simulink model "Citation_FlightGear_v2"  (R2026a)
settings: Solver=ode5  StopTime=40  FixedStep=0.01  EnableMultiTasking=on
InitFcn:
  | run('initcit.m')
  | run('id_init.m')
values from neighbouring files (symbols this model uses):
  cv1 = 20000    [gear_params.m]
  cv2 = cv1    (= 20000)    [gear_params.m]
  cv3 = 4000    [gear_params.m]
  cv4 = 20000    [gear_params.m]
  deltagmax1 = 0.25    [gear_params.m]
  deltagmax2 = deltagmax1    (= 0.25)    [gear_params.m]
  deltagmax3 = 0.24    [gear_params.m]
  deltagmax4 = 0.02    [gear_params.m]
  kt1 = 525020    [gear_params.m]
  kt2 = kt1    (= 525020)    [gear_params.m]
  kt3 = 457050    [gear_params.m]
  murol = 0.03*10    (= 0.3)    [gear_params.m]
  P1 = 2000    [gear_params.m]
  P2 = P1    (= 2000)    [gear_params.m]
  P3 = 2550    [gear_params.m]
  P4 = 40000    [gear_params.m]
  PL0 = 10000*eye(6)    [id_init.m]
  PM0 = 10000*eye(4)    [id_init.m]
  PN0 = 10000*eye(6)    [id_init.m]
  PX0 = 10000*eye(5)    [id_init.m]
  PY0 = 10000*eye(6)    [id_init.m]
  PZ0 = 10000*eye(4)    [id_init.m]
  thetaL0 = zeros(6,1)    [id_init.m]
  thetaM0 = zeros(4,1)    [id_init.m]
  thetaN0 = zeros(6,1)    [id_init.m]
  thetaX0 = zeros(5,1)    [id_init.m]
  thetaY0 = zeros(6,1)    [id_init.m]
  thetaZ0 = zeros(4,1)    [id_init.m]
  TL = 7.0875e-06    [id_init.m]    (also in plot_comparison_step_4.m = T_var(4))
  TM = 3.2564e-06    [id_init.m]    (also in plot_comparison_step_4.m = T_var(5))
  TN = 5.4692e-07    [id_init.m]    (also in plot_comparison_step_4.m = T_var(6))
  TX = 2.2784e-06    [id_init.m]    (also in plot_comparison_step_4.m = T_var(1))
  TY = 8.0633e-07    [id_init.m]    (also in plot_comparison_step_4.m = T_var(2))
  TZ = 2.8004e-05    [id_init.m]    (also in plot_comparison_step_4.m = T_var(3))
  xl1 = xcg-6.858    [gear_params.m]
  xl2 = xcg-6.858    [gear_params.m]
  xl3 = xcg-2.0752    [gear_params.m]
  xl4 = xcg-12.742    [gear_params.m]
  yl1 = 1.918    [gear_params.m]
  yl2 = -1.918    [gear_params.m]
  yl3 = 0    [gear_params.m]
  yl4 = 0    [gear_params.m]
  zl1 = zcg-1.701    [gear_params.m]
  zl2 = zcg-1.701    [gear_params.m]
  zl3 = zcg-1.7488    [gear_params.m]
  zl4 = zcg-2.78    [gear_params.m]
undefined symbols (not defined in the file or in its folder): chord, Deng, ealphag, ealphas, g0, hDME, hGS, lh, massinit, matbuaf, matdaf, matdam, matdbbf, matdeaf, matdgaf, matdqaf, matduaf, matdwaw, matedhr, mateif, matelhr, matemhr, matemv1, matemv2, matemve, matetam, mateuaf, matfaaf, matfaxl, matff, matibaf, matibb, matibmh, matipaf, matipmh, matiraf, matiuaf, matiwaf, matlaf, matlam, matleaf, matleam, matlgaf, matlqaf, matluaf, matmaaf, matmaam, matmaf, matmam, matmbbf, matmeaf, matmeam, matmgaf, matmqaf, matmrbr, matn1d, matn2d, matnbab, matnbaf, matnbmh ... (+53)
libraries: simulink x12, aerolibfltsims x3, aerolibconvert2 x2, aerolibobsolete x1, aerolibanimutils x1
(part 5 of 5)

== system Citation_FlightGear_v2/Cessna Citation 500/Citation model DASMAT/AIRCRAFT MODEL/EFM/Engmod/Citation eng_mod/Subsystem1/JT15 Dynamic1/Subsystem/engine/Gasgenerator ==
  note: N2 feedback
  note: N2dot
  PBCP : Inport
  he : Inport  Port=2
  sqrt(theta2) : Inport  Port=3
  Droop : Lookup  InputValues=[0 100]  Table="[0.1  2]"
  Fcn : Fcn  Expr=u[1]/u[2]
  Fcn1 : Fcn  Expr=u[1]/u[2]
  Governor : Product  InputSameDT=on  SaturateOnIntegerOverflow=on  OutDataTypeStr=Inherit: Same as first input
  Max accel : Subsystem  mask(Max Value){}
      mask help:
      | Output is maximum value of inputs.
      | y=max(u1,u2)
      mask Help: The Max block produces as output the maximum value of two scalars or vectors. If the inputs are vectors, the output will be a vector containing the maximum elements of the vectors.
      mask Display: disp('Max')
  Min accel : Subsystem  mask(Min Value){}
      mask help:
      | Output is minimum value of inputs.
      | y=min(u1,u2)
      mask Help: The Min block produces as output the minimum value of two scalars or vectors. If the inputs are vectors, the output will be a vector containing the minimum elements of the vectors.
      mask Display: disp('Min')
  Mux : Mux  Inputs=2
  Mux1 : Mux  Inputs=2
  N2 state : Integrator  InitialCondition=xt0(1)
  N2D : Lookup2D  RowIndex=matn2d(2:10,1)  ColumnIndex=matn2d(1,2:10)  Table=matn2d(2:10,2:10)
  Sum : Sum  Inputs=+-  InputSameDT=on  SaturateOnIntegerOverflow=on  OutDataTypeStr=Inherit: Same as first input
  fN2max : Lookup  InputValues=[25 40 70 94]  Table=[0 3 8 10]
  fN2min : Lookup  InputValues="[25     50   60   94 100]"  Table="[-0.05  -0.05    -2    -20 -28]"
  ft2FL : Gain  Gain=.01  SaturateOnIntegerOverflow=on  OutDataTypeStr=Inherit: Same as input  ParamDataTypeStr=Inherit: Same as input
  m2ft : Gain  Gain=(1/0.3048)  SaturateOnIntegerOverflow=on  OutDataTypeStr=Inherit: Same as input  ParamDataTypeStr=Inherit: Same as input
  N2 : Outport
  N2c : Outport  Port=2
  N2cdem : Outport  Port=3
  wires:
  sqrt(theta2)/1 -> Mux1/2, Mux/2
  N2D/1 -> Mux/1, Droop/1, Sum/1
  Fcn1/1 -> N2c/1
  Fcn/1 -> N2cdem/1
  Mux1/1 -> Fcn1/1
  Mux/1 -> Fcn/1
  Min accel/1(out_1) -> Max accel/1(in_1)
  ft2FL/1 -> N2D/2
  m2ft/1 -> ft2FL/1
  he/1 -> m2ft/1
  N2 state/1 -> Mux1/1, fN2min/1, fN2max/1, Sum/2, N2/1
  fN2max/1 -> Min accel/2(in_2)
  fN2min/1 -> Max accel/2(in_2)
  PBCP/1 -> N2D/1
  Droop/1 -> Governor/1
  Sum/1 -> Governor/2
  Governor/1 -> Min accel/1(in_1)
  Max accel/1(out_1) -> N2 state/1

== system Citation_FlightGear_v2/Cessna Citation 500/Citation model DASMAT/AIRCRAFT MODEL/EFM/Engmod/Citation eng_mod/Subsystem1/JT15 Dynamic/Subsystem/engine/Fan/Max accel ==
  in_1 : Inport
  in_2 : Inport  Port=2
  Sum : Sum  Inputs=-+  InputSameDT=on  SaturateOnIntegerOverflow=on  OutDataTypeStr=Inherit: Same as first input
  Switch : Switch
  out_1 : Outport
  wires:
  in_1/1 -> Sum/1, Switch/1
  in_2/1 -> Sum/2, Switch/3
  Sum/1 -> Switch/2
  Switch/1 -> out_1/1

== system Citation_FlightGear_v2/Cessna Citation 500/Citation model DASMAT/AIRCRAFT MODEL/EFM/Engmod/Citation eng_mod/Subsystem1/JT15 Dynamic/Subsystem/engine/Fan/Max decel ==
  in_1 : Inport
  in_2 : Inport  Port=2
  Sum : Sum  Inputs=+-  InputSameDT=on  SaturateOnIntegerOverflow=on  OutDataTypeStr=Inherit: Same as first input
  Switch : Switch
  out_1 : Outport
  wires:
  Switch/1 -> out_1/1
  Sum/1 -> Switch/2
  in_2/1 -> Sum/2, Switch/3
  in_1/1 -> Sum/1, Switch/1

== system Citation_FlightGear_v2/Cessna Citation 500/Citation model DASMAT/AIRCRAFT MODEL/EFM/Engmod/Citation eng_mod/Subsystem1/JT15 Dynamic/Subsystem/engine/Gasgenerator/Max accel ==
  in_1 : Inport
  in_2 : Inport  Port=2
  Sum : Sum  Inputs=+-  InputSameDT=on  SaturateOnIntegerOverflow=on  OutDataTypeStr=Inherit: Same as first input
  Switch : Switch
  out_1 : Outport
  wires:
  Switch/1 -> out_1/1
  Sum/1 -> Switch/2
  in_2/1 -> Sum/2, Switch/3
  in_1/1 -> Sum/1, Switch/1

== system Citation_FlightGear_v2/Cessna Citation 500/Citation model DASMAT/AIRCRAFT MODEL/EFM/Engmod/Citation eng_mod/Subsystem1/JT15 Dynamic/Subsystem/engine/Gasgenerator/Min accel ==
  in_1 : Inport
  in_2 : Inport  Port=2
  Sum : Sum  Inputs=-+  InputSameDT=on  SaturateOnIntegerOverflow=on  OutDataTypeStr=Inherit: Same as first input
  Switch : Switch
  out_1 : Outport
  wires:
  in_1/1 -> Sum/1, Switch/1
  in_2/1 -> Sum/2, Switch/3
  Sum/1 -> Switch/2
  Switch/1 -> out_1/1

== system Citation_FlightGear_v2/Cessna Citation 500/Citation model DASMAT/AIRCRAFT MODEL/EFM/Engmod/Citation eng_mod/Subsystem1/JT15 Dynamic1/Subsystem/engine/Fan/Max accel ==
  in_1 : Inport
  in_2 : Inport  Port=2
  Sum : Sum  Inputs=-+  InputSameDT=on  SaturateOnIntegerOverflow=on  OutDataTypeStr=Inherit: Same as first input
  Switch : Switch
  out_1 : Outport
  wires:
  in_1/1 -> Sum/1, Switch/1
  in_2/1 -> Sum/2, Switch/3
  Sum/1 -> Switch/2
  Switch/1 -> out_1/1

== system Citation_FlightGear_v2/Cessna Citation 500/Citation model DASMAT/AIRCRAFT MODEL/EFM/Engmod/Citation eng_mod/Subsystem1/JT15 Dynamic1/Subsystem/engine/Fan/Max decel ==
  in_1 : Inport
  in_2 : Inport  Port=2
  Sum : Sum  Inputs=+-  InputSameDT=on  SaturateOnIntegerOverflow=on  OutDataTypeStr=Inherit: Same as first input
  Switch : Switch
  out_1 : Outport
  wires:
  Switch/1 -> out_1/1
  Sum/1 -> Switch/2
  in_2/1 -> Sum/2, Switch/3
  in_1/1 -> Sum/1, Switch/1

== system Citation_FlightGear_v2/Cessna Citation 500/Citation model DASMAT/AIRCRAFT MODEL/EFM/Engmod/Citation eng_mod/Subsystem1/JT15 Dynamic1/Subsystem/engine/Gasgenerator/Max accel ==
  in_1 : Inport
  in_2 : Inport  Port=2
  Sum : Sum  Inputs=+-  InputSameDT=on  SaturateOnIntegerOverflow=on  OutDataTypeStr=Inherit: Same as first input
  Switch : Switch
  out_1 : Outport
  wires:
  Switch/1 -> out_1/1
  Sum/1 -> Switch/2
  in_2/1 -> Sum/2, Switch/3
  in_1/1 -> Sum/1, Switch/1

== system Citation_FlightGear_v2/Cessna Citation 500/Citation model DASMAT/AIRCRAFT MODEL/EFM/Engmod/Citation eng_mod/Subsystem1/JT15 Dynamic1/Subsystem/engine/Gasgenerator/Min accel ==
  in_1 : Inport
  in_2 : Inport  Port=2
  Sum : Sum  Inputs=-+  InputSameDT=on  SaturateOnIntegerOverflow=on  OutDataTypeStr=Inherit: Same as first input
  Switch : Switch
  out_1 : Outport
  wires:
  in_1/1 -> Sum/1, Switch/1
  in_2/1 -> Sum/2, Switch/3
  Sum/1 -> Switch/2
  Switch/1 -> out_1/1

== matlab function Citation_FlightGear_v2/RLS for CZ ==
  data: z input; theta_new output; phi input; theta_old input; P_old input; lambda input; reset input; P_new output; yhat output; innovation output
function [theta_new,P_new,yhat,innovation] = ...
    RLS_CZ(z,phi,theta_old,P_old,lambda,reset)

phi = phi(:);

% Previous covariance
Puse = P_old;

% Later used by Step 4
% Reset covariance, not parameter estimate
if reset > 0.5
    n = size(P_old,1);
    Puse = 10000*eye(n);
end

% Prediction using previous parameter estimate
yhat = phi.'*theta_old;

% Innovation
innovation = z - yhat;

% RLS gain
den = lambda + phi.'*Puse*phi;
K = (Puse*phi)/den;

% Parameter update
theta_new = theta_old + K*innovation;

% Covariance update
P_new = (Puse - K*(phi.'*Puse))/lambda;

% Remove numerical asymmetry
P_new = 0.5*(P_new + P_new.');

end

== matlab function Citation_FlightGear_v2/RLS for CL ==
  data: z input; theta_new output; phi input; theta_old input; P_old input; lambda input; reset input; P_new output; yhat output; innovation output
function [theta_new,P_new,yhat,innovation] = ...
    RLS_CL(z,phi,theta_old,P_old,lambda,reset)

phi = phi(:);

% Previous covariance
Puse = P_old;

% Later used by Step 4
% Reset covariance, not parameter estimate
if reset > 0.5
    n = size(P_old,1);
    Puse = 10000*eye(n);
end

% Prediction using previous parameter estimate
yhat = phi.'*theta_old;

% Innovation
innovation = z - yhat;

% RLS gain
den = lambda + phi.'*Puse*phi;
K = (Puse*phi)/den;

% Parameter update
theta_new = theta_old + K*innovation;

% Covariance update
P_new = (Puse - K*(phi.'*Puse))/lambda;

% Remove numerical asymmetry
P_new = 0.5*(P_new + P_new.');

end

== matlab function Citation_FlightGear_v2/RLS for Cm ==
  data: z input; theta_new output; phi input; theta_old input; P_old input; lambda input; reset input; P_new output; yhat output; innovation output
function [theta_new,P_new,yhat,innovation] = ...
    RLS_Cm(z,phi,theta_old,P_old,lambda,reset)

phi = phi(:);

% Previous covariance
Puse = P_old;

% Later used by Step 4
% Reset covariance, not parameter estimate
if reset > 0.5
    n = size(P_old,1);
    Puse = 10000*eye(n);
end

% Prediction using previous parameter estimate
yhat = phi.'*theta_old;

% Innovation
innovation = z - yhat;

% RLS gain
den = lambda + phi.'*Puse*phi;
K = (Puse*phi)/den;

% Parameter update
theta_new = theta_old + K*innovation;

% Covariance update
P_new = (Puse - K*(phi.'*Puse))/lambda;

% Remove numerical asymmetry
P_new = 0.5*(P_new + P_new.');

end

== matlab function Citation_FlightGear_v2/Monitoring/Monitoring Metrics ==
  data: innovations input; MA2 output; AUTOCORR output; VARIANCE output
function [MA2, AUTOCORR, VARIANCE] = monitor_metrics(innovations)
%#codegen

% Number of samples in monitoring window
N = 50;

% Lag used for autocorrelation
kgap = 5;

% Store previous innovation samples
persistent buffer count

if isempty(buffer)
    buffer = zeros(N,6);
    count = 0;
end

% Make sure innovations is a column vector
innovations = innovations(:);

% ---------------------------------------------------------
% Update buffer
% ---------------------------------------------------------

% Move all old values one position backwards
buffer(2:N,:) = buffer(1:N-1,:);

% Put newest innovations at the top
buffer(1,:) = innovations.';

if count < N
    count = count + 1;
end

% Initialize outputs
MA2      = zeros(6,1);
AUTOCORR = zeros(6,1);
VARIANCE = zeros(6,1);

% Do not calculate statistics until buffer is full
if count < N
    return;
end

% ---------------------------------------------------------
% Calculate metrics independently for X,Y,Z,L,M,N
% ---------------------------------------------------------

for j = 1:6

    e = buffer(:,j);

    % 1. Moving average of squared innovation
    MA2(j) = sum(e.^2)/N;

    % 2. Mean innovation
    e_mean = sum(e)/N;

    % 3. Variance
    VARIANCE(j) = sum((e - e_mean).^2)/(N-1);

    % 4. Autocorrelation at lag kgap
    AUTOCORR(j) = ...
        sum(e(1:N-kgap).*e(1+kgap:N))/N;

end

end

== matlab function Citation_FlightGear_v2/CIC lambda_CX ==
  data: z input; lambda_ad output; phi input; theta_old input; P_old input; Sigma0 input; lambda_min input; e output
function [lambda_ad,e] = CIC_lambda( ...
    z,phi,theta_old,P_old,Sigma0,lambda_min)

%#codegen

phi = phi(:);

% Prediction error / innovation
e = z - phi.'*theta_old;

% Information term
s = phi.'*P_old*phi;

% Constant Information Content forgetting factor
lambda_raw = 1 - e^2/(Sigma0*(1 + s));

% Numerical safety
lambda_ad = min(1.0,max(lambda_min,lambda_raw));

end

== matlab function Citation_FlightGear_v2/CIC lambda_CY ==
  data: z input; lambda_ad output; phi input; theta_old input; P_old input; Sigma0 input; lambda_min input; e output
function [lambda_ad,e] = CIC_lambda( ...
    z,phi,theta_old,P_old,Sigma0,lambda_min)

%#codegen

phi = phi(:);

% Prediction error / innovation
e = z - phi.'*theta_old;

% Information term
s = phi.'*P_old*phi;

% Constant Information Content forgetting factor
lambda_raw = 1 - e^2/(Sigma0*(1 + s));

% Numerical safety
lambda_ad = min(1.0,max(lambda_min,lambda_raw));

end

== matlab function Citation_FlightGear_v2/CIC lambda_CZ ==
  data: z input; lambda_ad output; phi input; theta_old input; P_old input; Sigma0 input; lambda_min input; e output
function [lambda_ad,e] = CIC_lambda( ...
    z,phi,theta_old,P_old,Sigma0,lambda_min)

%#codegen

phi = phi(:);

% Prediction error / innovation
e = z - phi.'*theta_old;

% Information term
s = phi.'*P_old*phi;

% Constant Information Content forgetting factor
lambda_raw = 1 - e^2/(Sigma0*(1 + s));

% Numerical safety
lambda_ad = min(1.0,max(lambda_min,lambda_raw));

end

== matlab function Citation_FlightGear_v2/CIC lambda_Cl ==
  data: z input; lambda_ad output; phi input; theta_old input; P_old input; Sigma0 input; lambda_min input; e output
function [lambda_ad,e] = CIC_lambda( ...
    z,phi,theta_old,P_old,Sigma0,lambda_min)

%#codegen

phi = phi(:);

% Prediction error / innovation
e = z - phi.'*theta_old;

% Information term
s = phi.'*P_old*phi;

% Constant Information Content forgetting factor
lambda_raw = 1 - e^2/(Sigma0*(1 + s));

% Numerical safety
lambda_ad = min(1.0,max(lambda_min,lambda_raw));

end

== matlab function Citation_FlightGear_v2/CIC lambda_Cm ==
  data: z input; lambda_ad output; phi input; theta_old input; P_old input; Sigma0 input; lambda_min input; e output
function [lambda_ad,e] = CIC_lambda( ...
    z,phi,theta_old,P_old,Sigma0,lambda_min)

%#codegen

phi = phi(:);

% Prediction error / innovation
e = z - phi.'*theta_old;

% Information term
s = phi.'*P_old*phi;

% Constant Information Content forgetting factor
lambda_raw = 1 - e^2/(Sigma0*(1 + s));

% Numerical safety
lambda_ad = min(1.0,max(lambda_min,lambda_raw));

end

== matlab function Citation_FlightGear_v2/CIC lambda_Cn ==
  data: z input; lambda_ad output; phi input; theta_old input; P_old input; Sigma0 input; lambda_min input; e output
function [lambda_ad,e] = CIC_lambda( ...
    z,phi,theta_old,P_old,Sigma0,lambda_min)

%#codegen

phi = phi(:);

% Prediction error / innovation
e = z - phi.'*theta_old;

% Information term
s = phi.'*P_old*phi;

% Constant Information Content forgetting factor
lambda_raw = 1 - e^2/(Sigma0*(1 + s));

% Numerical safety
lambda_ad = min(1.0,max(lambda_min,lambda_raw));

end

== matlab function Citation_FlightGear_v2/Regressors Symmetr. and Asymmetr. F//M Coefficients ==
  data: alpha input; beta input; p input; q input; r input; V input; de input; da input; dr input; phiX output; phiZM output; phiLat output
function [phiX,phiZM,phiLat] = ...
    build_regressors(alpha,beta,p,q,r,V,de,da,dr)

% Aircraft geometry
b = 13.3250;
c = 1.9910;

% Dimensionless angular-rate terms
qhat = q*c/V;
phat = p*b/(2*V);
rhat = r*b/(2*V);

% CX
phiX = [1;
        alpha;
        alpha^2;
        qhat;
        de];

% CZ and Cm
phiZM = [1;
         alpha;
         qhat;
         de];

% CY, Cl and Cn
phiLat = [1;
          beta;
          phat;
          rhat;
          da;
          dr];

end

== matlab function Citation_FlightGear_v2/Calculation of Force//Moments Coefficients ==
  data: p input; CX output; q input; r input; pdot input; qdot input; rdot input; V input; h input; anxb input; anyb input; anzb input; CY output; CZ output; Cl output; Cm output; Cn output; rho output
function [CX,CY,CZ,Cl,Cm,Cn,rho] = ...
    aero_measurements(p,q,r,pdot,qdot,rdot,V,h,anxb,anyb,anzb)

% Aircraft constants
m   = 4500;

Ixx = 11187.8;
Iyy = 22854.8;
Izz = 31974.8;
Ixz = 1930.1;

S = 24.9900;
b = 13.3250;
c = 1.9910;

% Atmosphere
g0     = 9.80665;
R      = 287.05;
lambda = -0.0065;
T0     = 288.15;
rho0   = 1.225;
htrop  = 11000;

% Density
Ttrop = T0 + lambda*htrop;

rho_trop = rho0 * (1 + lambda*htrop/T0)^(-g0/(R*lambda)-1);

if h <= htrop
    rho = rho0 * (1 + lambda*h/T0)^(-g0/(R*lambda)-1);
else
    rho = rho_trop * exp(-g0*(h-htrop)/(R*Ttrop));
end

% Convert specific forces from g to m/s^2
Ax = anxb*g0;
Ay = anyb*g0;
Az = anzb*g0;

% Dynamic pressure
qbar = 0.5*rho*V^2;

% Force coefficients
CX = m*Ax/(qbar*S);
CY = m*Ay/(qbar*S);
CZ = m*Az/(qbar*S);

% Aerodynamic moments from rigid-body rotational equations
L = Ixx*pdot + q*r*(Izz-Iyy) - (p*q + rdot)*Ixz;

M = Iyy*qdot + r*p*(Ixx-Izz) + (p^2-r^2)*Ixz;

N = Izz*rdot + p*q*(Iyy-Ixx) + (q*r-pdot)*Ixz;

% Moment coefficients
Cl = L/(qbar*S*b);
Cm = M/(qbar*S*c);
Cn = N/(qbar*S*b);

end

== matlab function Citation_FlightGear_v2/RLS for Cn ==
  data: z input; theta_new output; phi input; theta_old input; P_old input; lambda input; reset input; P_new output; yhat output; innovation output
function [theta_new,P_new,yhat,innovation] = ...
    RLS_Cn(z,phi,theta_old,P_old,lambda,reset)

phi = phi(:);

% Previous covariance
Puse = P_old;

% Later used by Step 4
% Reset covariance, not parameter estimate
if reset > 0.5
    n = size(P_old,1);
    Puse = 10000*eye(n);
end

% Prediction using previous parameter estimate
yhat = phi.'*theta_old;

% Innovation
innovation = z - yhat;

% RLS gain
den = lambda + phi.'*Puse*phi;
K = (Puse*phi)/den;

% Parameter update
theta_new = theta_old + K*innovation;

% Covariance update
P_new = (Puse - K*(phi.'*Puse))/lambda;

% Remove numerical asymmetry
P_new = 0.5*(P_new + P_new.');

end

== matlab function Citation_FlightGear_v2/RLS for CX ==
  data: z input; theta_new output; phi input; theta_old input; P_old input; lambda input; reset input; P_new output; yhat output; innovation output
function [theta_new,P_new,yhat,innovation] = ...
    RLS_CX(z,phi,theta_old,P_old,lambda,reset)

phi = phi(:);

% Previous covariance
Puse = P_old;

% Later used by Step 4
% Reset covariance, not parameter estimate
if reset > 0.5
    n = size(P_old,1);
    Puse = 10000*eye(n);
end

% Prediction using previous parameter estimate
yhat = phi.'*theta_old;

% Innovation
innovation = z - yhat;

% RLS gain
den = lambda + phi.'*Puse*phi;
K = (Puse*phi)/den;

% Parameter update
theta_new = theta_old + K*innovation;

% Covariance update
P_new = (Puse - K*(phi.'*Puse))/lambda;

% Remove numerical asymmetry
P_new = 0.5*(P_new + P_new.');

end

== matlab function Citation_FlightGear_v2/RLS for CY ==
  data: z input; theta_new output; phi input; theta_old input; P_old input; lambda input; reset input; P_new output; yhat output; innovation output
function [theta_new,P_new,yhat,innovation] = ...
    RLS_CY(z,phi,theta_old,P_old,lambda,reset)

phi = phi(:);

% Previous covariance
Puse = P_old;

% Later used by Step 4
% Reset covariance, not parameter estimate
if reset > 0.5
    n = size(P_old,1);
    Puse = 10000*eye(n);
end

% Prediction using previous parameter estimate
yhat = phi.'*theta_old;

% Innovation
innovation = z - yhat;

% RLS gain
den = lambda + phi.'*Puse*phi;
K = (Puse*phi)/den;

% Parameter update
theta_new = theta_old + K*innovation;

% Covariance update
P_new = (Puse - K*(phi.'*Puse))/lambda;

% Remove numerical asymmetry
P_new = 0.5*(P_new + P_new.');

end
